simulink model "Button_detection_Storage_B"  (R2015b)
settings: Solver=VariableStepAuto  StartTime=0.0  StopTime=10.0  RelTol=1e-3
settings Model: Creator=Roberto91  LastModifiedBy=Andrea

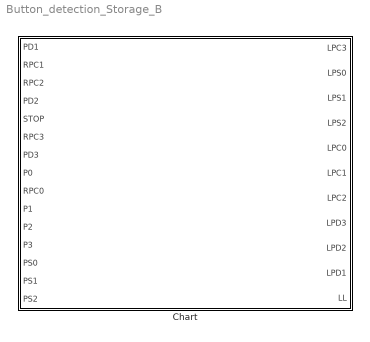
== system Button_detection_Storage_B ==
  Chart : Stateflow chart  TreatAsAtomicUnit=on

== stateflow chart Button_detection_Storage_B/Chart ==
  state Save_energy
    en:
    LL=not(Q_LL);
  state Timer_LL
    state Set_tmr
      en:
      Q_LL=true;
    state Counting
      en:
      ET_LL= ET_LL + 1;
      Q_LL=false;
    state Set
      en:
      IN_LL=true;
      PT_LL=10;
    (junction 264) -> Timer_LL.Set_tmr [order 1] : [ET_LL==PT_LL]
    Timer_LL.Set_tmr -> (junction 265)
    Timer_LL.Counting -> (junction 264)
    (junction 264) -> (junction 265) [order 2]
    (default) -> Timer_LL.Set
    Timer_LL.Set -> (junction 266)
    (junction 266) -> Timer_LL.Counting [order 1] : [ET_LL<PT_LL]
    (junction 266) -> (junction 265) [order 2]
  state BUTTON_DOWN
    state Button_DOWN_1
      en:
      BUTTON_DOWN(2)=true;
      BUT_TEMP=1;
      LPD1=true;
      PUSHED=true;
      UPDATE=false;
      IN_LL=false; ET_LL=0;
    state First_but_1
      en:
      BUT_1=BUT_TEMP;
      FIRST_BUT=false;
    state No_button_pushed
    state Button_DOWN_2
      en:
      BUTTON_DOWN(3)=true;
      BUT_TEMP=2;
      LPD2=true;
      PUSHED=true;
      UPDATE=false;
      IN_LL=false; ET_LL=0;
    state First_but_2
      en:
      BUT_1=BUT_TEMP;
      FIRST_BUT=false;
    state Button_DOWN_3
      en:
      BUTTON_DOWN(4)=true;
      BUT_TEMP=3;
      LPD3=true;
      PUSHED=true;
      UPDATE=false;
      IN_LL=false; ET_LL=0;
    state First_but_3
      en:
      BUT_1=BUT_TEMP;
      FIRST_BUT=false;
    BUTTON_DOWN.No_button_pushed -> (junction 358)
    (junction 358) -> Button_DOWN_1 [order 1] : [PD1]
    Button_DOWN_1 -> (junction 359)
    (junction 359) -> BUTTON_DOWN.First_but_1 [order 1] : [FIRST_BUT && not(RPC1)]
    BUTTON_DOWN.First_but_1 -> (junction 360)
    (default) -> BUTTON_DOWN.No_button_pushed
    (junction 358) -> (junction 361) [order 2]
    (junction 359) -> (junction 362) [order 2]
    (junction 360) -> (junction 363)
    (junction 362) -> (junction 361)
    (junction 363) -> (junction 362)
    (junction 361) -> (junction 364)
    (junction 364) -> Button_DOWN_2 [order 1] : [PD2]
    Button_DOWN_2 -> (junction 365)
    (junction 365) -> BUTTON_DOWN.First_but_2 [order 1] : [FIRST_BUT && not(RPC2)]
    BUTTON_DOWN.First_but_2 -> (junction 366)
    (junction 364) -> (junction 367) [order 2]
    (junction 365) -> (junction 368) [order 2]
    (junction 366) -> (junction 369)
    (junction 368) -> (junction 367)
    (junction 369) -> (junction 368)
    (junction 367) -> (junction 370)
    (junction 370) -> Button_DOWN_3 [order 1] : [PD3]
    Button_DOWN_3 -> (junction 371)
    (junction 371) -> BUTTON_DOWN.First_but_3 [order 1] : [FIRST_BUT && not(RPC3)]
    BUTTON_DOWN.First_but_3 -> (junction 372)
    (junction 370) -> (junction 373) [order 2]
    (junction 371) -> (junction 374) [order 2]
    (junction 372) -> (junction 375)
    (junction 374) -> (junction 373)
    (junction 375) -> (junction 374)
  state BUTTON_CAR
    state Button_CAR_0
      en:
      BUTTON_CAR(1)=true;
      BUT_TEMP=0;
      LPC0=true;
      PUSHED=true;
      UPDATE=false;
      IN_LL=false; ET_LL=0;
    state First_but_0
      en:
      BUT_1=BUT_TEMP;
      FIRST_BUT=false;
    state NO_operation
    state First_but_01
      en:
      BUT_1_CAR=BUT_TEMP;
      FIRST_BUT_CAR=false;
    state Button_CAR_1
      en:
      BUTTON_CAR(2)=true;
      BUT_TEMP=1;
      LPC1=true;
      PUSHED=true;
      UPDATE=false;
      IN_LL=false; ET_LL=0;
    state First_but_1
      en:
      BUT_1=BUT_TEMP;
      FIRST_BUT=false;
    state First_but_02
      en:
      BUT_1_CAR=BUT_TEMP;
      FIRST_BUT_CAR=false;
    state Button_CAR_2
      en:
      BUTTON_CAR(3)=true;
      BUT_TEMP=2;
      LPC2=true;
      PUSHED=true;
      UPDATE=false;
      IN_LL=false; ET_LL=0;
    state First_but_2
      en:
      BUT_1=BUT_TEMP;
      FIRST_BUT=false;
    state First_but_03
      en:
      BUT_1_CAR=BUT_TEMP;
      FIRST_BUT_CAR=false;
    state Button_CAR_3
      en:
      BUTTON_CAR(4)=true;
      BUT_TEMP=3;
      LPC3=true;
      PUSHED=true;
      UPDATE=false;
      IN_LL=false; ET_LL=0;
    state First_but_3
      en:
      BUT_1=BUT_TEMP;
      FIRST_BUT=false;
    state First_but_04
      en:
      BUT_1_CAR=BUT_TEMP;
      FIRST_BUT_CAR=false;
    state Start
      en:	 START=true;
      BUT_1_CAR=FLOOR;
      FIRST_BUT_CAR=true;
    (junction 283) -> Button_CAR_0 [order 1] : [P0]
    Button_CAR_0 -> (junction 284)
    (junction 284) -> BUTTON_CAR.First_but_0 [order 1] : [FIRST_BUT && not(RPC0)]
    BUTTON_CAR.First_but_0 -> (junction 285)
    BUTTON_CAR.NO_operation -> (junction 283)
    (default) -> BUTTON_CAR.NO_operation
    (junction 283) -> (junction 286) [order 2]
    (junction 284) -> (junction 287) [order 2]
    (junction 285) -> (junction 288)
    (junction 288) -> (junction 287)
    (junction 287) -> (junction 417)
    (junction 417) -> First_but_01 [order 1] : [FIRST_BUT_CAR && not(RPC0)]
    First_but_01 -> (junction 418)
    (junction 417) -> (junction 419) [order 2]
    (junction 418) -> (junction 416)
    (junction 419) -> (junction 286)
    (junction 416) -> (junction 419)
    (junction 286) -> (junction 291)
    Button_CAR_1 -> (junction 289)
    (junction 289) -> BUTTON_CAR.First_but_1 [order 1] : [FIRST_BUT && not(RPC1)]
    BUTTON_CAR.First_but_1 -> (junction 290)
    (junction 289) -> (junction 293) [order 2]
    (junction 290) -> (junction 294)
    (junction 291) -> Button_CAR_1 [order 1] : [P1]
    (junction 291) -> (junction 292) [order 2]
    (junction 294) -> (junction 293)
    (junction 293) -> (junction 429)
    (junction 429) -> First_but_02 [order 1] : [FIRST_BUT_CAR && not(RPC1)]
    First_but_02 -> (junction 430)
    (junction 429) -> (junction 431) [order 2]
    (junction 430) -> (junction 428)
    (junction 431) -> (junction 292)
    (junction 428) -> (junction 431)
    (junction 292) -> (junction 295)
    (junction 295) -> Button_CAR_2 [order 1] : [P2]
    Button_CAR_2 -> (junction 296)
    (junction 296) -> BUTTON_CAR.First_but_2 [order 1] : [FIRST_BUT && not(RPC2)]
    BUTTON_CAR.First_but_2 -> (junction 297)
    (junction 295) -> (junction 298) [order 2]
    (junction 296) -> (junction 299) [order 2]
    (junction 297) -> (junction 300)
    (junction 300) -> (junction 299)
    (junction 299) -> (junction 441)
    (junction 441) -> First_but_03 [order 1] : [FIRST_BUT_CAR && not(RPC2)]
    First_but_03 -> (junction 442)
    (junction 441) -> (junction 443) [order 2]
    (junction 442) -> (junction 440)
    (junction 443) -> (junction 298)
    (junction 440) -> (junction 443)
    (junction 298) -> (junction 301)
    (junction 301) -> Button_CAR_3 [order 1] : [P3]
    Button_CAR_3 -> (junction 302)
    (junction 302) -> BUTTON_CAR.First_but_3 [order 1] : [FIRST_BUT && not(RPC3)]
    BUTTON_CAR.First_but_3 -> (junction 303)
    (junction 301) -> (junction 304) [order 2]
    (junction 302) -> (junction 305) [order 2]
    (junction 303) -> (junction 306)
    (junction 306) -> (junction 305)
    (junction 305) -> (junction 453)
    (junction 453) -> First_but_04 [order 1] : [FIRST_BUT_CAR && not(RPC3)]
    First_but_04 -> (junction 454)
    (junction 453) -> (junction 455) [order 2]
    (junction 454) -> (junction 452)
    (junction 455) -> (junction 304)
    (junction 452) -> (junction 455)
    (junction 304) -> (junction 473)
    Start -> (junction 477)
    (junction 473) -> Start [order 1] : [not(BUTTON_CAR(1) || BUTTON_CAR(2) || BUTTON_CAR(3) || BUTTON_CAR(4))]
    (junction 473) -> (junction 479) [order 2]
    (junction 477) -> (junction 481)
    (junction 481) -> (junction 479)
  state BUTTON_UP
    state Button_UP_0
      en:
      BUTTON_UP(1)=true;
      BUT_TEMP=0;
      LPS0=true;
      PUSHED=true;
      UPDATE=false;
      IN_LL=false; ET_LL=0;
    state First_but_0
      en:
      BUT_1=BUT_TEMP;
      FIRST_BUT=false;
    state No_button_pushed
    state Button_UP_1
      en:
      BUTTON_UP(2)=true;
      BUT_TEMP=1;
      LPS1=true;
      PUSHED=true;
      UPDATE=false;
      IN_LL=false; ET_LL=0;
    state First_but_1
      en:
      BUT_1=BUT_TEMP;
      FIRST_BUT=false;
    state Button_UP_2
      en:
      BUTTON_UP(3)=true;
      BUT_TEMP=2;
      LPS2=true;
      PUSHED=true;
      UPDATE=false;
      IN_LL=false; ET_LL=0;
    state First_but_2
      en:
      BUT_1=BUT_TEMP;
      FIRST_BUT=false;
    (default) -> BUTTON_UP.No_button_pushed
    BUTTON_UP.No_button_pushed -> (junction 62)
    (junction 62) -> Button_UP_0 [order 1] : [PS0]
    Button_UP_0 -> (junction 63)
    (junction 63) -> BUTTON_UP.First_but_0 [order 1] : [FIRST_BUT && not(RPC0)]
    BUTTON_UP.First_but_0 -> (junction 64)
    (junction 62) -> (junction 67) [order 2]
    (junction 63) -> (junction 65) [order 2]
    (junction 64) -> (junction 66)
    (junction 66) -> (junction 65)
    (junction 65) -> (junction 67)
    (junction 67) -> (junction 68)
    (junction 68) -> Button_UP_1 [order 1] : [PS1]
    Button_UP_1 -> (junction 69)
    (junction 69) -> BUTTON_UP.First_but_1 [order 1] : [FIRST_BUT && not(RPC1)]
    BUTTON_UP.First_but_1 -> (junction 70)
    (junction 68) -> (junction 71) [order 2]
    (junction 69) -> (junction 72) [order 2]
    (junction 70) -> (junction 73)
    (junction 72) -> (junction 71)
    (junction 73) -> (junction 72)
    (junction 71) -> (junction 75)
    BUTTON_UP.First_but_2 -> (junction 74)
    (junction 74) -> (junction 79)
    (junction 75) -> Button_UP_2 [order 1] : [PS2]
    Button_UP_2 -> (junction 76)
    (junction 76) -> BUTTON_UP.First_but_2 [order 1] : [FIRST_BUT && not(RPC2)]
    (junction 75) -> (junction 77) [order 2]
    (junction 76) -> (junction 78) [order 2]
    (junction 78) -> (junction 77)
    (junction 79) -> (junction 78)
  state Max_Min_assignment
    state NO_operation
    state Min_but
      en:
      BUTTON=MIN_BUT;
    state Max_but
      en:
      BUTTON=MAX_BUT;
    state Button1_car
      en: BUTTON=BUT_1_CAR;
    state First_but
      en:
      BUTTON=BUT_1;
    state Max_but1
      en:
      MAX_BUT=2;
    state Max_but2
      en:
      MAX_BUT=1;
    state Max_but3
      en:
      MAX_BUT=0;
    state Min_but1
      en:
      MIN_BUT=1;
    state Min_but2
      en:
      MIN_BUT=2;
    state Min_but3
      en:
      MIN_BUT=3;
    state MAX
      en:
      MAX_BUT=BUT_TEMP;
    state MIN
      en:
      MIN_BUT=BUT_TEMP;
    state Set_motion
      en: MOTION=1;
      START=false;
    state Max0
      en:MAX_BUT=0;
    state Updating_button_0
      en:
      BUTTON=MAX_BUT;
    state Set_motion0
      en: MOTION=0;
      START=false;
    state Min3
      en: MIN_BUT=3;
    state Updating_button_1
      en:
      BUTTON=MIN_BUT;
    (junction 117) -> Min_but [order 1] : [(MAX_BUT-FLOOR)>(FLOOR-MIN_BUT) && (FIRST_BUT_CAR)]
    Min_but -> (junction 118)
    (junction 119) -> (junction 117) [order 1] : [not(FLAG_STOP) && MOTION==2 && FLAG==3]
    Max_Min_assignment.NO_operation -> (junction 119)
    (default) -> Max_Min_assignment.NO_operation
    (junction 117) -> (junction 120) [order 2]
    (junction 118) -> (junction 121)
    (junction 119) -> (junction 122) [order 2]
    (junction 120) -> Max_but [order 1] : [(MAX_BUT-FLOOR)<(FLOOR-MIN_BUT) && (FIRST_BUT_CAR)]
    Max_but -> (junction 121)
    (junction 121) -> (junction 493)
    (junction 120) -> (junction 489) [order 2]
    (junction 489) -> Button1_car [order 1] : [not(FIRST_BUT_CAR)]
    Button1_car -> (junction 493)
    (junction 493) -> (junction 124)
    (junction 489) -> First_but [order 2]
    First_but -> (junction 123)
    (junction 124) -> (junction 123)
    (junction 123) -> (junction 122)
    (junction 122) -> (junction 125)
    (junction 125) -> (junction 126) [order 1] : [BUTTON==FLOOR && FLAG==3]
    (junction 126) -> (junction 127) [order 1] : [MOTION==0]
        | {MOTION=1;
        | UPDATE=true;}
    (junction 127) -> Max_but1 [order 1] : [BUTTON_UP(2)]
    Max_but1 -> (junction 128)
    (junction 125) -> (junction 139) [order 2]
    (junction 126) -> (junction 131) [order 2]
    (junction 127) -> (junction 129) [order 2]
    (junction 128) -> (junction 130)
    (junction 129) -> Max_but2 [order 1] : [BUTTON_UP(1)]
    Max_but2 -> (junction 130)
    (junction 129) -> Max_but3 [order 2]
    (junction 130) -> (junction 133)
    Max_but3 -> (junction 132)
    (junction 132) -> (junction 131)
    (junction 133) -> (junction 132)
    (junction 131) -> (junction 134)
    (junction 134) -> (junction 135) [order 1] : [MOTION==1]
        | {MOTION=0;
        | UPDATE=true;}
    (junction 135) -> Min_but1 [order 1] : [BUTTON_DOWN(1)]
    Min_but1 -> (junction 136)
    (junction 134) -> (junction 140) [order 2]
    (junction 135) -> (junction 137) [order 2]
    (junction 136) -> (junction 138)
    (junction 137) -> Min_but2 [order 1] : [BUTTON_DOWN(2)]
    Min_but2 -> (junction 138)
    (junction 137) -> Min_but3 [order 2]
    (junction 138) -> (junction 142)
    Min_but3 -> (junction 141)
    (junction 140) -> (junction 139)
    (junction 141) -> (junction 140)
    (junction 142) -> (junction 141)
    (junction 139) -> (junction 144)
    (junction 144) -> (junction 145) [order 1] : [PUSHED]
    (junction 145) -> (junction 146) [order 1] : [not(BUT_TEMP==FLOOR) || not(MOTION==2)]
    (junction 146) -> MAX [order 1] : [MAX_BUT<BUT_TEMP && not(UPDATE)]
    MAX -> (junction 143)
    (junction 144) -> (junction 158) [order 2]
    (junction 145) -> (junction 151) [order 2]
    (junction 146) -> (junction 147) [order 2]
    (junction 143) -> (junction 148)
    (junction 148) -> (junction 147)
    (junction 147) -> (junction 149)
    (junction 149) -> MIN [order 1] : [MIN_BUT>BUT_TEMP && not(UPDATE)]
    MIN -> (junction 150)
    (junction 149) -> (junction 152) [order 2]
    (junction 150) -> (junction 153)
    (junction 152) -> (junction 151)
    (junction 153) -> (junction 152)
    (junction 151) -> (junction 154)
    (junction 499) -> Set_motion [order 1] : [BUT_1_CAR<BUT_1 && START && FLAG==3 && (BUTTON_CAR(1) || BUTTON_CAR(2) || BUTTON_CAR(3) || BUTTON_CAR(4))]
    Set_motion -> (junction 502)
    (junction 502) -> Max0 [order 1] : [BUT_1==MAX_BUT]
    Max0 -> (junction 155)
    (junction 154) -> (junction 499) [order 1] : [MOTION==0]
    (junction 502) -> (junction 155) [order 2]
    (junction 155) -> (junction 509)
    (junction 154) -> (junction 156) [order 2]
    (junction 499) -> Updating_button_0 [order 2]
    Updating_button_0 -> (junction 509)
    (junction 509) -> (junction 527)
    (junction 513) -> Set_motion0 [order 1] : [BUT_1_CAR<BUT_1 && START && FLAG==3 && (BUTTON_CAR(1) || BUTTON_CAR(2) || BUTTON_CAR(3) || BUTTON_CAR(4))]
    Set_motion0 -> (junction 517)
    (junction 517) -> Min3 [order 1] : [BUT_1==MIN_BUT]
    Min3 -> (junction 527)
    (junction 156) -> (junction 513) [order 1] : [MOTION==1]
    (junction 517) -> (junction 527) [order 2]
    (junction 527) -> (junction 523)
    (junction 513) -> Updating_button_1 [order 2]
    (junction 156) -> (junction 159) [order 2]
    Updating_button_1 -> (junction 523)
    (junction 523) -> (junction 160)
    (junction 159) -> (junction 158)
    (junction 160) -> (junction 159)
  state GoTo_PositionControl
    en:
    BUTTON=BUT_TEMP;
    FLAG=2;
  state Emergency
    en:
    FLAG_EMG=true;
    FLAG=4;
  state Timer_EME
    state Set_tmr
      en:
      Q_EME=true;
    state Counting
      en:
      ET_EME= ET_EME + 1;
      Q_EME=false;
    state Set
      en:
      IN_EME=true;
      PT_EME=3;
    (junction 249) -> Timer_EME.Set_tmr [order 1] : [ET_EME==PT_EME]
    Timer_EME.Set_tmr -> (junction 250)
    Timer_EME.Counting -> (junction 249)
    (junction 249) -> (junction 250) [order 2]
    (default) -> Timer_EME.Set
    Timer_EME.Set -> (junction 251)
    (junction 251) -> Timer_EME.Counting [order 1] : [ET_EME<PT_EME]
    (junction 251) -> (junction 250) [order 2]
  state Not_Emergency
    en:
    IN_EME=false;
    ET_EME=0;
  state SwitchingOFF_LEDs
    en:
    LPD3=false;
    LPD2=false;
    LPS2=false;
    LPD1=false;
    LPS1=false;
    LPS0=false;
  (default) -> (junction 412)
  (junction 412) -> (junction 279) [order 1] : [FLAG==1 && not(PUSHED)]
      | {BUTTON=FLOOR;
      | BUT_TEMP=BUTTON;
      | BUT_1=FLOOR;
      | BUT_1_CAR=FLOOR;
      | FIRST_BUT=true;
      | FIRST_BUT_CAR=true;}
  (junction 279) -> Timer_LL [order 1] : [not(FLAG_STOP)]
  Timer_LL -> Save_energy
  Save_energy -> (junction 413)
  (junction 279) -> (junction 281) [order 2]
  (junction 412) -> (junction 280) [order 2]
  (junction 413) -> (junction 356)
  (junction 281) -> (junction 280)
  (junction 356) -> (junction 281)
  (junction 280) -> BUTTON_CAR
  BUTTON_UP -> BUTTON_DOWN
  BUTTON_DOWN -> Max_Min_assignment
  Max_Min_assignment -> (junction 414)
  BUTTON_CAR -> BUTTON_UP
  (junction 414) -> (junction 58)
  (junction 58) -> (junction 415)
  (junction 415) -> (junction 1)
  (junction 1) -> (junction 4) [order 1] : [FLAG==1]
  (junction 4) -> GoTo_PositionControl [order 1] : [PUSHED]
  GoTo_PositionControl -> (junction 2)
  (junction 1) -> (junction 25) [order 2]
  (junction 4) -> (junction 5) [order 2]
  (junction 2) -> (junction 7)
  (junction 7) -> (junction 5)
  (junction 5) -> (junction 6)
  Emergency -> (junction 3)
  (junction 6) -> Timer_EME [order 1] : [STOP]
      | {IN_LL=false; ET_LL=0;FLAG=1;}
  Timer_EME -> (junction 9)
  (junction 9) -> Emergency [order 1] : [Q_EME]
  (junction 3) -> (junction 11)
  (junction 6) -> Not_Emergency [order 2]
  (junction 9) -> (junction 10) [order 2]
  (junction 11) -> (junction 10)
  (junction 10) -> (junction 28)
  Not_Emergency -> (junction 28)
  SwitchingOFF_LEDs -> (junction 8)
  (junction 28) -> SwitchingOFF_LEDs [order 1] : [FLAG_STOP && FLAG==2]
  (junction 8) -> (junction 57)
  (junction 28) -> (junction 26) [order 2]
  (junction 26) -> (junction 25)
  (junction 57) -> (junction 26)
  data: IN_EME local =false; FLAG_EMG local =false; LPC3 output =false; LPS0 output =false; LPS1 output =false; LPS2 output =false; LPC0 output =false; LPC1 output =false; LPC2 output =false; LPD3 output =false; LPD2 output =false; IN_LL local =false; LPD1 output =false; LL output =false; PT_EME local =0; Q_EME local =false; ET_EME local =0; MOTION local =2; BUT_1 local =0; START local =false; FLAG local =0; MAX_BUT local =0; BUTTON local =0; MIN_BUT local =3; PT_LL local =0; BUT_TEMP local =0; PUSHED local =false; UPDATE local; Q_LL local =false; ET_LL local =0; FIRST_BUT_CAR local =false; BUT_1_CAR local =0; BUTTON_UP local size=[1,4] =[false,false,false,false]; BUTTON_DOWN local size=[1,4] =[false,false,false,false]; FIRST_BUT local =false; BUTTON_CAR local size=[1,4] =[false,false,false,false]; FLOOR local =0; PD1 input boolean; RPC1 input; RPC2 input; PD2 input boolean; STOP input; RPC3 input; PD3 input boolean; P0 input boolean; RPC0 input; P1 input boolean; P2 input boolean; P3 input boolean; PS0 input boolean; PS1 input boolean; PS2 input boolean; FLAG_STOP local =false
